simulink model "Project1"  (R2022b)
settings: Solver=VariableStepAuto  StartTime=0.0  StopTime=10.0  RelTol=1e-3
undefined symbols (not defined in the file): a, b, c
libraries: simulink x15
settings Model: Creator=ROYAN  LastModifiedBy=ROYAN

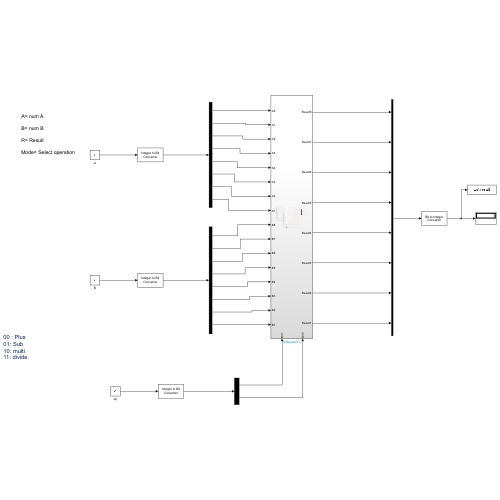
[thumbnail: Simulink's stored preview of the top-level diagram]
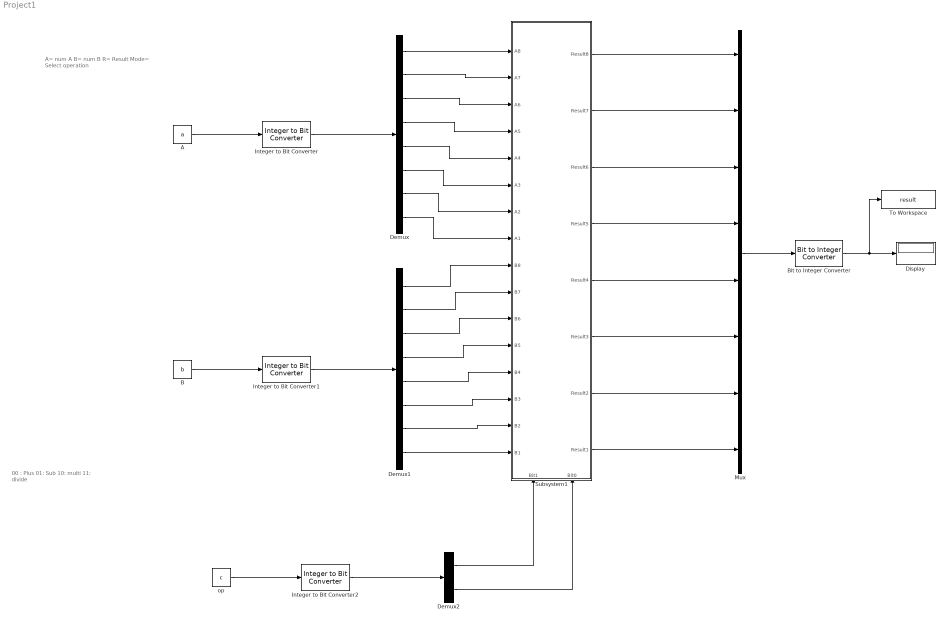
== system Project1 ==
  note: 00 : Plus
      | 01: Sub
      | 10: multi
      | 11: divide
  note: A= num A
      |
      | B= num B
      |
      | R= Result
      |
      | Mode= Select operation
  A : Constant  Value=a
  B : Constant  Value=b
  Bit to Integer Converter : simulink/Logic and Bit Operations/Bit to Integer Converter  nbits=8  bitOrder=MSB first  signedOutputValues=Signed  outDtype=Inherit via internal rule  outDtypeSigned=Inherit via internal rule
  Demux : Demux  Outputs=8
  Demux1 : Demux  Outputs=8
  Demux2 : Demux  Outputs=2
  Display : Display
  Integer to Bit Converter : simulink/Logic and Bit Operations/Integer to Bit Converter  nbits=8  signedInputValues=Unsigned  bitOrder=MSB first  outDtype=Inherit via internal rule
  Integer to Bit Converter1 : simulink/Logic and Bit Operations/Integer to Bit Converter  nbits=8  signedInputValues=Unsigned  bitOrder=MSB first  outDtype=Inherit via internal rule
  Integer to Bit Converter2 : simulink/Logic and Bit Operations/Integer to Bit Converter  nbits=2  signedInputValues=Unsigned  bitOrder=MSB first  outDtype=Inherit via internal rule
  Mux : Mux  Inputs=8
  Subsystem1 : Subsystem
      settings: PortSchema="{\"entries\":[{\"content\":{\"sides\":[{\"content\":{\"connectorIds\":[\"In1\",\"In2\",\"In3\",\"In4\",\"In5\",\"In6\",\"In7\",\"In8\",\"In9\",\"In10\",\"In11\",\"In12\",\"In13\",\"In14\",\"In15\",\"In16\"]},\"type\":\"ConnectorPlacement.EquallySpacedRectSide\",\"uuid\":\"3d59707f-8e10-42d7-a8bb-d15e440eb3d5\"},{\"content\":{\"connectorIds\":[\"Out1\",\"Out2\",\"Out3\",\"Out4\",\"Out5\",\"Out6\",\"Out7\",\"Out8\"],\"side\":\"RIGHT\"},\"type\":\"ConnectorPlacement.EquallySpacedRectSide\",\"uuid\":\"1a8263b8-a282-4efb-b962-f7f661c6be06\"},{\"content\":{\"connectorIds\":[],\"side\":\"TOP\"},\"type\":\"ConnectorPlacement.EquallySpacedRectSide\",\"uuid\":\"6e97006b-dc23-4e30-9819-71647844af05\"},{\"content\":{\"connectorIds\":[\"In17\",\"In18\"],\"side\":\"BOTTOM\"},\"type\":\"ConnectorPlacement.EquallySpacedRectSide\",\"uuid\":\"8a081856-ff6f-46be-8c16-ac5173067d34\"}]},\"type\":\"ConnectorPlacement.EquallySpacedConnector\",\"uuid\":\"19aafbc0-9711-4025-9e66-34128d3b56ae\"}],\"packageUris\":[\"http://schema.mathworks.com/mf0/Connector/R2020b\"],\"version\":\"1.0\"}"
  To Workspace : ToWorkspace  VariableName=result  SampleTime=-1
  op : Constant  Value=c
  wires:
  Subsystem1/1(Result8) -> Mux/1
  Subsystem1/2(Result7) -> Mux/2
  Subsystem1/3(Result6) -> Mux/3
  Subsystem1/4(Result5) -> Mux/4
  Subsystem1/7(Result2) -> Mux/7
  Subsystem1/8(Result1) -> Mux/8
  Subsystem1/6(Result3) -> Mux/6
  Subsystem1/5(Result4) -> Mux/5
  B/1 -> Integer to Bit Converter1/1
  Demux1/8 -> Subsystem1/16(B1)
  Demux1/7 -> Subsystem1/15(B2)
  Demux1/6 -> Subsystem1/14(B3)
  Demux1/5 -> Subsystem1/13(B4)
  Demux1/4 -> Subsystem1/12(B5)
  Mux/1 -> Bit to Integer Converter/1
  Bit to Integer Converter/1 -> To Workspace/1, Display/1
  Integer to Bit Converter1/1 -> Demux1/1
  Demux/1 -> Subsystem1/1(A8)
  Demux/2 -> Subsystem1/2(A7)
  Demux/3 -> Subsystem1/3(A6)
  Demux/4 -> Subsystem1/4(A5)
  Demux/5 -> Subsystem1/5(A4)
  Demux/6 -> Subsystem1/6(A3)
  Demux/7 -> Subsystem1/7(A2)
  Demux/8 -> Subsystem1/8(A1)
  Demux1/3 -> Subsystem1/11(B6)
  Demux1/1 -> Subsystem1/9(B8)
  Demux1/2 -> Subsystem1/10(B7)
  Integer to Bit Converter/1 -> Demux/1
  A/1 -> Integer to Bit Converter/1
  Integer to Bit Converter2/1 -> Demux2/1
  op/1 -> Integer to Bit Converter2/1
  Demux2/1 -> Subsystem1/17(Bit1)
  Demux2/2 -> Subsystem1/18(Bit0)

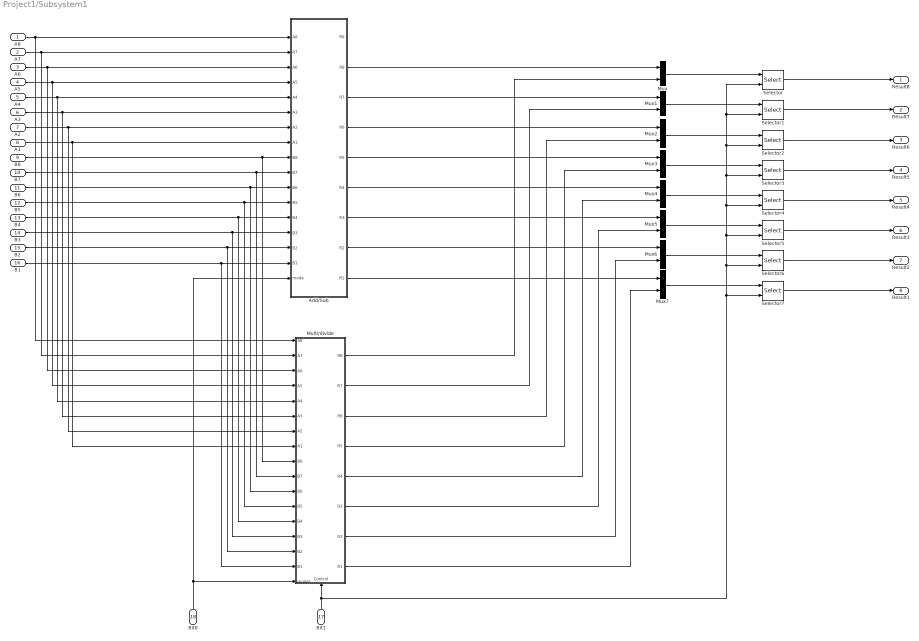
== system Project1/Subsystem1 ==
  A8 : Inport
  A7 : Inport  Port=2
  A6 : Inport  Port=3
  A5 : Inport  Port=4
  A4 : Inport  Port=5
  A3 : Inport  Port=6
  A2 : Inport  Port=7
  A1 : Inport  Port=8
  B8 : Inport  Port=9
  B7 : Inport  Port=10
  B6 : Inport  Port=11
  B5 : Inport  Port=12
  B4 : Inport  Port=13
  B3 : Inport  Port=14
  B2 : Inport  Port=15
  B1 : Inport  Port=16
  Bit1 : Inport  Port=17
  Bit0 : Inport  Port=18
  Add/Sub : Subsystem
  "Multi/divide " : Subsystem
      settings: PortSchema="{\"entries\":[{\"content\":{\"sides\":[{\"content\":{\"connectorIds\":[\"In1\",\"In2\",\"In3\",\"In4\",\"In5\",\"In6\",\"In7\",\"In8\",\"In9\",\"In10\",\"In11\",\"In12\",\"In13\",\"In14\",\"In15\",\"In16\",\"In17\"]},\"type\":\"ConnectorPlacement.EquallySpacedRectSide\",\"uuid\":\"d787903a-2fc8-4344-b2b5-b1474f8fa836\"},{\"content\":{\"connectorIds\":[\"Out1\",\"Out2\",\"Out3\",\"Out4\",\"Out5\",\"Out6\",\"Out7\",\"Out8\"],\"side\":\"RIGHT\"},\"type\":\"ConnectorPlacement.EquallySpacedRectSide\",\"uuid\":\"e4051a45-32f8-4700-a673-fbaf13b5a8eb\"},{\"content\":{\"connectorIds\":[],\"side\":\"TOP\"},\"type\":\"ConnectorPlacement.EquallySpacedRectSide\",\"uuid\":\"26f5a230-4be8-43df-bd8c-ec355ee08860\"},{\"content\":{\"connectorIds\":[\"In18\"],\"side\":\"BOTTOM\"},\"type\":\"ConnectorPlacement.EquallySpacedRectSide\",\"uuid\":\"cbf4e858-912e-4040-9d22-8fbb14c5758f\"}]},\"type\":\"ConnectorPlacement.EquallySpacedConnector\",\"uuid\":\"a4b69b5f-bd5b-46ed-959e-11d2f0394428\"}],\"packageUris\":[\"http://schema.mathworks.com/mf0/Connector/R2020b\"],\"version\":\"1.0\"}"
  Mux{,1..7} (8 alike) : Mux  Inputs=2
  Selector{,1..7} (8 alike) : Selector  NumberOfDimensions=2  IndexMode=Zero-based  InputPortWidth=3  IndexOptions=Select all,Index vector (port)  Indices=[1 3],1  OutputSizes=1,1
  Result8 : Outport
  Result7 : Outport  Port=2
  Result6 : Outport  Port=3
  Result5 : Outport  Port=4
  Result4 : Outport  Port=5
  Result3 : Outport  Port=6
  Result2 : Outport  Port=7
  Result1 : Outport  Port=8
  wires:
  A8/1 -> "Multi/divide "/1(A8), Add/Sub/1(A8)
  A7/1 -> "Multi/divide "/2(A7), Add/Sub/2(A7)
  A6/1 -> "Multi/divide "/3(A6), Add/Sub/3(A6)
  A5/1 -> "Multi/divide "/4(A5), Add/Sub/4(A5)
  A4/1 -> "Multi/divide "/5(A4), Add/Sub/5(A4)
  A3/1 -> "Multi/divide "/6(A3), Add/Sub/6(A3)
  A2/1 -> "Multi/divide "/7(A2), Add/Sub/7(A2)
  A1/1 -> "Multi/divide "/8(A1), Add/Sub/8(A1)
  B8/1 -> "Multi/divide "/9(B8), Add/Sub/9(B8)
  B7/1 -> "Multi/divide "/10(B7), Add/Sub/10(B7)
  B6/1 -> "Multi/divide "/11(B6), Add/Sub/11(B6)
  B5/1 -> "Multi/divide "/12(B5), Add/Sub/12(B5)
  B4/1 -> "Multi/divide "/13(B4), Add/Sub/13(B4)
  B3/1 -> "Multi/divide "/14(B3), Add/Sub/14(B3)
  B2/1 -> "Multi/divide "/15(B2), Add/Sub/15(B2)
  B1/1 -> "Multi/divide "/16(B1), Add/Sub/16(B1)
  Bit0/1 -> Add/Sub/17(mode), "Multi/divide "/17(mode1)
  Mux/1 -> Selector/1
  Selector/1 -> Result8/1
  Bit1/1 -> "Multi/divide "/18(Control), Selector6/2, Selector1/2, Selector/2, Selector2/2, Selector3/2, Selector4/2, Selector5/2, Selector7/2
  Selector1/1 -> Result7/1
  Mux1/1 -> Selector1/1
  Mux2/1 -> Selector2/1
  Selector2/1 -> Result6/1
  Mux3/1 -> Selector3/1
  Selector3/1 -> Result5/1
  Selector4/1 -> Result4/1
  Mux4/1 -> Selector4/1
  Mux5/1 -> Selector5/1
  Selector5/1 -> Result3/1
  Mux7/1 -> Selector7/1
  Mux6/1 -> Selector6/1
  Selector6/1 -> Result2/1
  Selector7/1 -> Result1/1
  Add/Sub/2(R8) -> Mux/1
  "Multi/divide "/1(R8) -> Mux/2
  Add/Sub/3(R7) -> Mux1/1
  "Multi/divide "/2(R7) -> Mux1/2
  Add/Sub/4(R6) -> Mux2/1
  "Multi/divide "/3(R6) -> Mux2/2
  Add/Sub/5(R5) -> Mux3/1
  "Multi/divide "/4(R5) -> Mux3/2
  Add/Sub/6(R4) -> Mux4/1
  "Multi/divide "/5(R4) -> Mux4/2
  Add/Sub/7(R3) -> Mux5/1
  "Multi/divide "/6(R3) -> Mux5/2
  Add/Sub/8(R2) -> Mux6/1
  "Multi/divide "/7(R2) -> Mux6/2
  Add/Sub/9(R1) -> Mux7/1
  "Multi/divide "/8(R1) -> Mux7/2

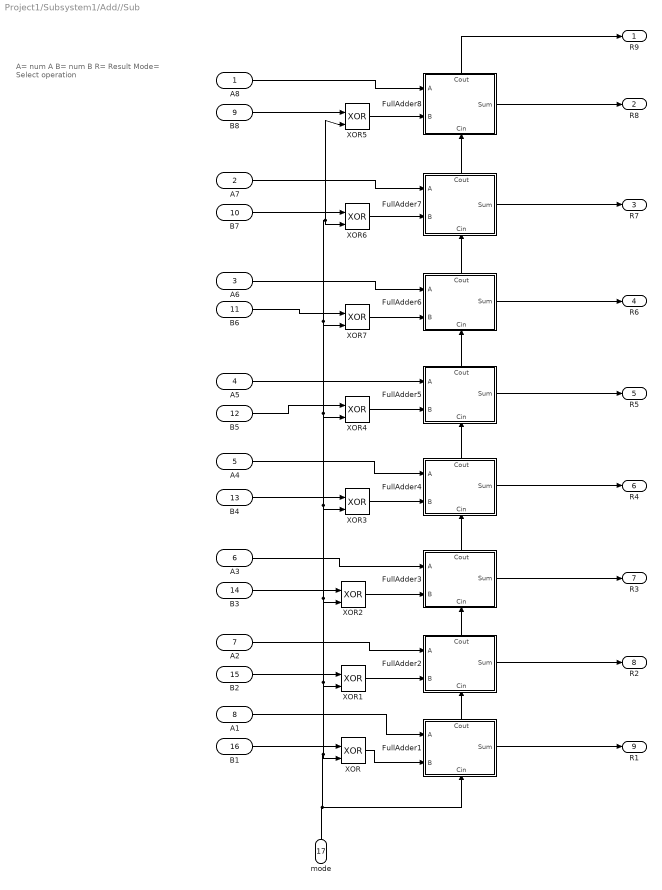
== system Project1/Subsystem1/Add//Sub ==
  note: A= num A
      |
      | B= num B
      |
      | R= Result
      |
      | Mode= Select operation
  A8 : Inport
  A7 : Inport  Port=2
  A6 : Inport  Port=3
  A5 : Inport  Port=4
  A4 : Inport  Port=5
  A3 : Inport  Port=6
  A2 : Inport  Port=7
  A1 : Inport  Port=8
  B8 : Inport  Port=9
  B7 : Inport  Port=10
  B6 : Inport  Port=11
  B5 : Inport  Port=12
  B4 : Inport  Port=13
  B3 : Inport  Port=14
  B2 : Inport  Port=15
  B1 : Inport  Port=16
  mode : Inport  Port=17
  FullAdder1 : Subsystem
      settings: PortSchema="{\"entries\":[{\"content\":{\"sides\":[{\"content\":{\"connectorIds\":[\"In1\",\"In2\"]},\"type\":\"ConnectorPlacement.EquallySpacedRectSide\",\"uuid\":\"fe566a19-caaa-40f2-a564-acf59556d540\"},{\"content\":{\"connectorIds\":[\"Out1\"],\"side\":\"RIGHT\"},\"type\":\"ConnectorPlacement.EquallySpacedRectSide\",\"uuid\":\"72e5ab5f-929d-480e-bf59-fcaf5ea21c8f\"},{\"content\":{\"connectorIds\":[\"Out2\"],\"side\":\"TOP\"},\"type\":\"ConnectorPlacement.EquallySpacedRectSide\",\"uuid\":\"fa7afc02-c581-4624-b2e4-f0b490a4f45a\"},{\"content\":{\"connectorIds\":[\"In3\"],\"side\":\"BOTTOM\"},\"type\":\"ConnectorPlacement.EquallySpacedRectSide\",\"uuid\":\"7004099e-9eda-49bf-b4e1-5ef4db972604\"}]},\"type\":\"ConnectorPlacement.EquallySpacedConnector\",\"uuid\":\"f3081cfd-4ff5-48bf-a714-5b2ae9791e36\"}],\"packageUris\":[\"http://schema.mathworks.com/mf0/Connector/R2020b\"],\"version\":\"1.0\"}"
  FullAdder2 : Subsystem
      settings: PortSchema="{\"entries\":[{\"content\":{\"sides\":[{\"content\":{\"connectorIds\":[\"In1\",\"In2\"]},\"type\":\"ConnectorPlacement.EquallySpacedRectSide\",\"uuid\":\"fe566a19-caaa-40f2-a564-acf59556d540\"},{\"content\":{\"connectorIds\":[\"Out1\"],\"side\":\"RIGHT\"},\"type\":\"ConnectorPlacement.EquallySpacedRectSide\",\"uuid\":\"72e5ab5f-929d-480e-bf59-fcaf5ea21c8f\"},{\"content\":{\"connectorIds\":[\"Out2\"],\"side\":\"TOP\"},\"type\":\"ConnectorPlacement.EquallySpacedRectSide\",\"uuid\":\"fa7afc02-c581-4624-b2e4-f0b490a4f45a\"},{\"content\":{\"connectorIds\":[\"In3\"],\"side\":\"BOTTOM\"},\"type\":\"ConnectorPlacement.EquallySpacedRectSide\",\"uuid\":\"7004099e-9eda-49bf-b4e1-5ef4db972604\"}]},\"type\":\"ConnectorPlacement.EquallySpacedConnector\",\"uuid\":\"f3081cfd-4ff5-48bf-a714-5b2ae9791e36\"}],\"packageUris\":[\"http://schema.mathworks.com/mf0/Connector/R2020b\"],\"version\":\"1.0\"}"
  FullAdder3 : Subsystem
      settings: PortSchema="{\"entries\":[{\"content\":{\"sides\":[{\"content\":{\"connectorIds\":[\"In1\",\"In2\"]},\"type\":\"ConnectorPlacement.EquallySpacedRectSide\",\"uuid\":\"fe566a19-caaa-40f2-a564-acf59556d540\"},{\"content\":{\"connectorIds\":[\"Out1\"],\"side\":\"RIGHT\"},\"type\":\"ConnectorPlacement.EquallySpacedRectSide\",\"uuid\":\"72e5ab5f-929d-480e-bf59-fcaf5ea21c8f\"},{\"content\":{\"connectorIds\":[\"Out2\"],\"side\":\"TOP\"},\"type\":\"ConnectorPlacement.EquallySpacedRectSide\",\"uuid\":\"fa7afc02-c581-4624-b2e4-f0b490a4f45a\"},{\"content\":{\"connectorIds\":[\"In3\"],\"side\":\"BOTTOM\"},\"type\":\"ConnectorPlacement.EquallySpacedRectSide\",\"uuid\":\"7004099e-9eda-49bf-b4e1-5ef4db972604\"}]},\"type\":\"ConnectorPlacement.EquallySpacedConnector\",\"uuid\":\"f3081cfd-4ff5-48bf-a714-5b2ae9791e36\"}],\"packageUris\":[\"http://schema.mathworks.com/mf0/Connector/R2020b\"],\"version\":\"1.0\"}"
  FullAdder4 : Subsystem
      settings: PortSchema="{\"entries\":[{\"content\":{\"sides\":[{\"content\":{\"connectorIds\":[\"In1\",\"In2\"]},\"type\":\"ConnectorPlacement.EquallySpacedRectSide\",\"uuid\":\"fe566a19-caaa-40f2-a564-acf59556d540\"},{\"content\":{\"connectorIds\":[\"Out1\"],\"side\":\"RIGHT\"},\"type\":\"ConnectorPlacement.EquallySpacedRectSide\",\"uuid\":\"72e5ab5f-929d-480e-bf59-fcaf5ea21c8f\"},{\"content\":{\"connectorIds\":[\"Out2\"],\"side\":\"TOP\"},\"type\":\"ConnectorPlacement.EquallySpacedRectSide\",\"uuid\":\"fa7afc02-c581-4624-b2e4-f0b490a4f45a\"},{\"content\":{\"connectorIds\":[\"In3\"],\"side\":\"BOTTOM\"},\"type\":\"ConnectorPlacement.EquallySpacedRectSide\",\"uuid\":\"7004099e-9eda-49bf-b4e1-5ef4db972604\"}]},\"type\":\"ConnectorPlacement.EquallySpacedConnector\",\"uuid\":\"f3081cfd-4ff5-48bf-a714-5b2ae9791e36\"}],\"packageUris\":[\"http://schema.mathworks.com/mf0/Connector/R2020b\"],\"version\":\"1.0\"}"
  FullAdder5 : Subsystem
      settings: PortSchema="{\"entries\":[{\"content\":{\"sides\":[{\"content\":{\"connectorIds\":[\"In1\",\"In2\"]},\"type\":\"ConnectorPlacement.EquallySpacedRectSide\",\"uuid\":\"fe566a19-caaa-40f2-a564-acf59556d540\"},{\"content\":{\"connectorIds\":[\"Out1\"],\"side\":\"RIGHT\"},\"type\":\"ConnectorPlacement.EquallySpacedRectSide\",\"uuid\":\"72e5ab5f-929d-480e-bf59-fcaf5ea21c8f\"},{\"content\":{\"connectorIds\":[\"Out2\"],\"side\":\"TOP\"},\"type\":\"ConnectorPlacement.EquallySpacedRectSide\",\"uuid\":\"fa7afc02-c581-4624-b2e4-f0b490a4f45a\"},{\"content\":{\"connectorIds\":[\"In3\"],\"side\":\"BOTTOM\"},\"type\":\"ConnectorPlacement.EquallySpacedRectSide\",\"uuid\":\"7004099e-9eda-49bf-b4e1-5ef4db972604\"}]},\"type\":\"ConnectorPlacement.EquallySpacedConnector\",\"uuid\":\"f3081cfd-4ff5-48bf-a714-5b2ae9791e36\"}],\"packageUris\":[\"http://schema.mathworks.com/mf0/Connector/R2020b\"],\"version\":\"1.0\"}"
  FullAdder6 : Subsystem
      settings: PortSchema="{\"entries\":[{\"content\":{\"sides\":[{\"content\":{\"connectorIds\":[\"In1\",\"In2\"]},\"type\":\"ConnectorPlacement.EquallySpacedRectSide\",\"uuid\":\"fe566a19-caaa-40f2-a564-acf59556d540\"},{\"content\":{\"connectorIds\":[\"Out1\"],\"side\":\"RIGHT\"},\"type\":\"ConnectorPlacement.EquallySpacedRectSide\",\"uuid\":\"72e5ab5f-929d-480e-bf59-fcaf5ea21c8f\"},{\"content\":{\"connectorIds\":[\"Out2\"],\"side\":\"TOP\"},\"type\":\"ConnectorPlacement.EquallySpacedRectSide\",\"uuid\":\"fa7afc02-c581-4624-b2e4-f0b490a4f45a\"},{\"content\":{\"connectorIds\":[\"In3\"],\"side\":\"BOTTOM\"},\"type\":\"ConnectorPlacement.EquallySpacedRectSide\",\"uuid\":\"7004099e-9eda-49bf-b4e1-5ef4db972604\"}]},\"type\":\"ConnectorPlacement.EquallySpacedConnector\",\"uuid\":\"f3081cfd-4ff5-48bf-a714-5b2ae9791e36\"}],\"packageUris\":[\"http://schema.mathworks.com/mf0/Connector/R2020b\"],\"version\":\"1.0\"}"
  FullAdder7 : Subsystem
      settings: PortSchema="{\"entries\":[{\"content\":{\"sides\":[{\"content\":{\"connectorIds\":[\"In1\",\"In2\"]},\"type\":\"ConnectorPlacement.EquallySpacedRectSide\",\"uuid\":\"fe566a19-caaa-40f2-a564-acf59556d540\"},{\"content\":{\"connectorIds\":[\"Out1\"],\"side\":\"RIGHT\"},\"type\":\"ConnectorPlacement.EquallySpacedRectSide\",\"uuid\":\"72e5ab5f-929d-480e-bf59-fcaf5ea21c8f\"},{\"content\":{\"connectorIds\":[\"Out2\"],\"side\":\"TOP\"},\"type\":\"ConnectorPlacement.EquallySpacedRectSide\",\"uuid\":\"fa7afc02-c581-4624-b2e4-f0b490a4f45a\"},{\"content\":{\"connectorIds\":[\"In3\"],\"side\":\"BOTTOM\"},\"type\":\"ConnectorPlacement.EquallySpacedRectSide\",\"uuid\":\"7004099e-9eda-49bf-b4e1-5ef4db972604\"}]},\"type\":\"ConnectorPlacement.EquallySpacedConnector\",\"uuid\":\"f3081cfd-4ff5-48bf-a714-5b2ae9791e36\"}],\"packageUris\":[\"http://schema.mathworks.com/mf0/Connector/R2020b\"],\"version\":\"1.0\"}"
  FullAdder8 : Subsystem
      settings: PortSchema="{\"entries\":[{\"content\":{\"sides\":[{\"content\":{\"connectorIds\":[\"In1\",\"In2\"]},\"type\":\"ConnectorPlacement.EquallySpacedRectSide\",\"uuid\":\"fe566a19-caaa-40f2-a564-acf59556d540\"},{\"content\":{\"connectorIds\":[\"Out1\"],\"side\":\"RIGHT\"},\"type\":\"ConnectorPlacement.EquallySpacedRectSide\",\"uuid\":\"72e5ab5f-929d-480e-bf59-fcaf5ea21c8f\"},{\"content\":{\"connectorIds\":[\"Out2\"],\"side\":\"TOP\"},\"type\":\"ConnectorPlacement.EquallySpacedRectSide\",\"uuid\":\"fa7afc02-c581-4624-b2e4-f0b490a4f45a\"},{\"content\":{\"connectorIds\":[\"In3\"],\"side\":\"BOTTOM\"},\"type\":\"ConnectorPlacement.EquallySpacedRectSide\",\"uuid\":\"7004099e-9eda-49bf-b4e1-5ef4db972604\"}]},\"type\":\"ConnectorPlacement.EquallySpacedConnector\",\"uuid\":\"f3081cfd-4ff5-48bf-a714-5b2ae9791e36\"}],\"packageUris\":[\"http://schema.mathworks.com/mf0/Connector/R2020b\"],\"version\":\"1.0\"}"
  XOR{,1..7} (8 alike) : Logic  Operator=XOR  IconShape=distinctive  AllPortsSameDT=off  OutDataTypeStr=boolean
  R9 : Outport
  R8 : Outport  Port=2
  R7 : Outport  Port=3
  R6 : Outport  Port=4
  R5 : Outport  Port=5
  R4 : Outport  Port=6
  R3 : Outport  Port=7
  R2 : Outport  Port=8
  R1 : Outport  Port=9
  wires:
  FullAdder1/2(Cout) -> FullAdder2/3(Cin)
  FullAdder3/2(Cout) -> FullAdder4/3(Cin)
  A6/1 -> FullAdder6/1(A)
  FullAdder3/1(Sum) -> R3/1
  FullAdder6/2(Cout) -> FullAdder7/3(Cin)
  FullAdder5/2(Cout) -> FullAdder6/3(Cin)
  FullAdder1/1(Sum) -> R1/1
  A8/1 -> FullAdder8/1(A)
  FullAdder8/1(Sum) -> R8/1
  FullAdder5/1(Sum) -> R5/1
  A7/1 -> FullAdder7/1(A)
  A5/1 -> FullAdder5/1(A)
  FullAdder4/2(Cout) -> FullAdder5/3(Cin)
  FullAdder4/1(Sum) -> R4/1
  FullAdder6/1(Sum) -> R6/1
  A2/1 -> FullAdder2/1(A)
  FullAdder8/2(Cout) -> R9/1
  A4/1 -> FullAdder4/1(A)
  FullAdder2/1(Sum) -> R2/1
  FullAdder7/2(Cout) -> FullAdder8/3(Cin)
  A1/1 -> FullAdder1/1(A)
  A3/1 -> FullAdder3/1(A)
  FullAdder2/2(Cout) -> FullAdder3/3(Cin)
  FullAdder7/1(Sum) -> R7/1
  mode/1 -> XOR5/2, XOR6/2, XOR7/2, XOR4/2, XOR3/2, XOR2/2, XOR1/2, XOR/2, FullAdder1/3(Cin)
  B1/1 -> XOR/1
  XOR/1 -> FullAdder1/2(B)
  B2/1 -> XOR1/1
  XOR1/1 -> FullAdder2/2(B)
  B3/1 -> XOR2/1
  XOR2/1 -> FullAdder3/2(B)
  B4/1 -> XOR3/1
  XOR3/1 -> FullAdder4/2(B)
  B5/1 -> XOR4/1
  XOR4/1 -> FullAdder5/2(B)
  B6/1 -> XOR7/1
  XOR7/1 -> FullAdder6/2(B)
  B7/1 -> XOR6/1
  XOR6/1 -> FullAdder7/2(B)
  B8/1 -> XOR5/1
  XOR5/1 -> FullAdder8/2(B)

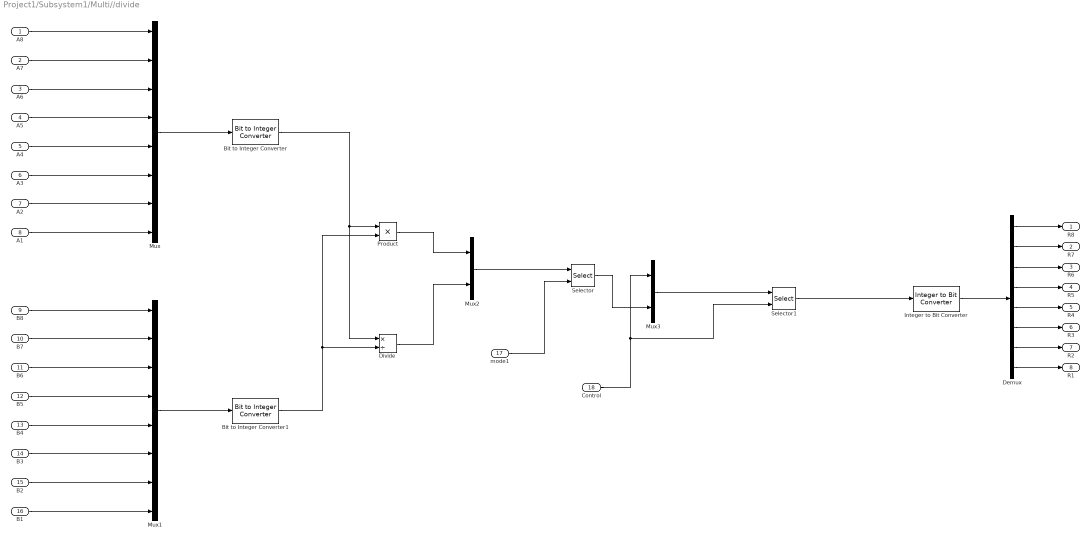
== system Project1/Subsystem1/Multi//divide  ==
  A8 : Inport
  A7 : Inport  Port=2
  A6 : Inport  Port=3
  A5 : Inport  Port=4
  A4 : Inport  Port=5
  A3 : Inport  Port=6
  A2 : Inport  Port=7
  A1 : Inport  Port=8
  B8 : Inport  Port=9
  B7 : Inport  Port=10
  B6 : Inport  Port=11
  B5 : Inport  Port=12
  B4 : Inport  Port=13
  B3 : Inport  Port=14
  B2 : Inport  Port=15
  B1 : Inport  Port=16
  mode1 : Inport  Port=17
  Control : Inport  Port=18
  Bit to Integer Converter : simulink/Logic and Bit Operations/Bit to Integer Converter  nbits=8  bitOrder=MSB first  signedOutputValues=Unsigned  outDtype=Inherit via internal rule  outDtypeSigned=Inherit via internal rule
  Bit to Integer Converter1 : simulink/Logic and Bit Operations/Bit to Integer Converter  nbits=8  bitOrder=MSB first  signedOutputValues=Unsigned  outDtype=Inherit via internal rule  outDtypeSigned=Inherit via internal rule
  Demux : Demux  Outputs=8
  Divide : Product  Inputs=*/
  Integer to Bit Converter : simulink/Logic and Bit Operations/Integer to Bit Converter  nbits=8  signedInputValues=Unsigned  bitOrder=MSB first  outDtype=Inherit via internal rule
  Mux : Mux  Inputs=8
  Mux1 : Mux  Inputs=8
  Mux2 : Mux  Inputs=2
  Mux3 : Mux  Inputs=2
  Product : Product
  Selector : Selector  NumberOfDimensions=2  IndexMode=Zero-based  InputPortWidth=3  IndexOptions=Select all,Index vector (port)  Indices=[1 3],1  OutputSizes=1,1
  Selector1 : Selector  NumberOfDimensions=2  IndexMode=Zero-based  InputPortWidth=3  IndexOptions=Select all,Index vector (port)  Indices=[1 3],1  OutputSizes=1,1
  R8 : Outport
  R7 : Outport  Port=2
  R6 : Outport  Port=3
  R5 : Outport  Port=4
  R4 : Outport  Port=5
  R3 : Outport  Port=6
  R2 : Outport  Port=7
  R1 : Outport  Port=8
  wires:
  A8/1 -> Mux/1
  A7/1 -> Mux/2
  A6/1 -> Mux/3
  A5/1 -> Mux/4
  A4/1 -> Mux/5
  A2/1 -> Mux/7
  A1/1 -> Mux/8
  A3/1 -> Mux/6
  Mux/1 -> Bit to Integer Converter/1
  Mux1/1 -> Bit to Integer Converter1/1
  B8/1 -> Mux1/1
  B7/1 -> Mux1/2
  B6/1 -> Mux1/3
  B5/1 -> Mux1/4
  B4/1 -> Mux1/5
  B3/1 -> Mux1/6
  B2/1 -> Mux1/7
  B1/1 -> Mux1/8
  Bit to Integer Converter/1 -> Divide/1, Product/1
  Bit to Integer Converter1/1 -> Product/2, Divide/2
  Product/1 -> Mux2/1
  Divide/1 -> Mux2/2
  mode1/1 -> Selector/2
  Mux2/1 -> Selector/1
  Integer to Bit Converter/1 -> Demux/1
  Demux/1 -> R8/1
  Demux/2 -> R7/1
  Demux/8 -> R1/1
  Demux/7 -> R2/1
  Demux/6 -> R3/1
  Demux/5 -> R4/1
  Demux/4 -> R5/1
  Demux/3 -> R6/1
  Control/1 -> Mux3/1, Selector1/2
  Selector1/1 -> Integer to Bit Converter/1
  Mux3/1 -> Selector1/1
  Selector/1 -> Mux3/2

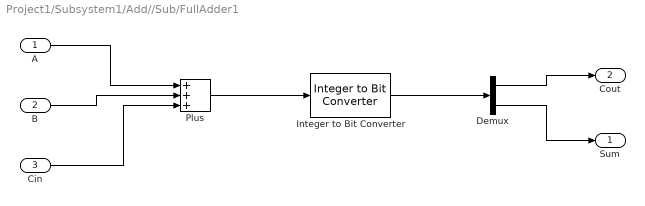
== system Project1/Subsystem1/Add//Sub/FullAdder1 ==
  A : Inport
  B : Inport  Port=2
  Cin : Inport  Port=3
  Demux : Demux  Outputs=2
  Integer to Bit Converter : simulink/Logic and Bit Operations/Integer to Bit Converter  nbits=2  signedInputValues=Unsigned  bitOrder=MSB first  outDtype=Inherit via internal rule
  Plus : Sum  Inputs=+++
  Sum : Outport
  Cout : Outport  Port=2
  wires:
  Demux/2 -> Sum/1
  Demux/1 -> Cout/1
  A/1 -> Plus/1
  Cin/1 -> Plus/3
  Plus/1 -> Integer to Bit Converter/1
  B/1 -> Plus/2
  Integer to Bit Converter/1 -> Demux/1

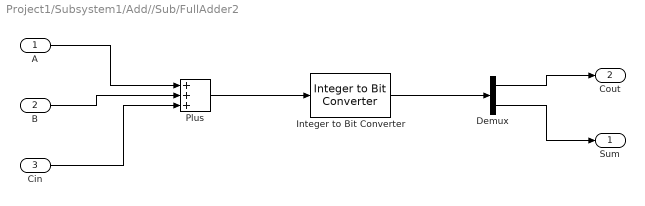
== system Project1/Subsystem1/Add//Sub/FullAdder2 ==
  A : Inport
  B : Inport  Port=2
  Cin : Inport  Port=3
  Demux : Demux  Outputs=2
  Integer to Bit Converter : simulink/Logic and Bit Operations/Integer to Bit Converter  nbits=2  signedInputValues=Unsigned  bitOrder=MSB first  outDtype=Inherit via internal rule
  Plus : Sum  Inputs=+++
  Sum : Outport
  Cout : Outport  Port=2
  wires:
  Demux/2 -> Sum/1
  Demux/1 -> Cout/1
  A/1 -> Plus/1
  Cin/1 -> Plus/3
  Plus/1 -> Integer to Bit Converter/1
  B/1 -> Plus/2
  Integer to Bit Converter/1 -> Demux/1

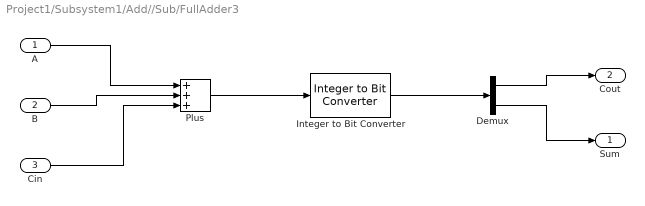
== system Project1/Subsystem1/Add//Sub/FullAdder3 ==
  A : Inport
  B : Inport  Port=2
  Cin : Inport  Port=3
  Demux : Demux  Outputs=2
  Integer to Bit Converter : simulink/Logic and Bit Operations/Integer to Bit Converter  nbits=2  signedInputValues=Unsigned  bitOrder=MSB first  outDtype=Inherit via internal rule
  Plus : Sum  Inputs=+++
  Sum : Outport
  Cout : Outport  Port=2
  wires:
  Integer to Bit Converter/1 -> Demux/1
  B/1 -> Plus/2
  Plus/1 -> Integer to Bit Converter/1
  Cin/1 -> Plus/3
  A/1 -> Plus/1
  Demux/1 -> Cout/1
  Demux/2 -> Sum/1

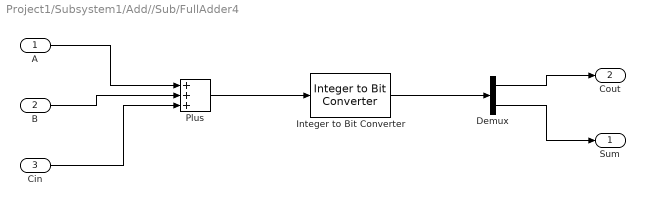
== system Project1/Subsystem1/Add//Sub/FullAdder4 ==
  A : Inport
  B : Inport  Port=2
  Cin : Inport  Port=3
  Demux : Demux  Outputs=2
  Integer to Bit Converter : simulink/Logic and Bit Operations/Integer to Bit Converter  nbits=2  signedInputValues=Unsigned  bitOrder=MSB first  outDtype=Inherit via internal rule
  Plus : Sum  Inputs=+++
  Sum : Outport
  Cout : Outport  Port=2
  wires:
  Demux/2 -> Sum/1
  Demux/1 -> Cout/1
  A/1 -> Plus/1
  Cin/1 -> Plus/3
  Plus/1 -> Integer to Bit Converter/1
  B/1 -> Plus/2
  Integer to Bit Converter/1 -> Demux/1

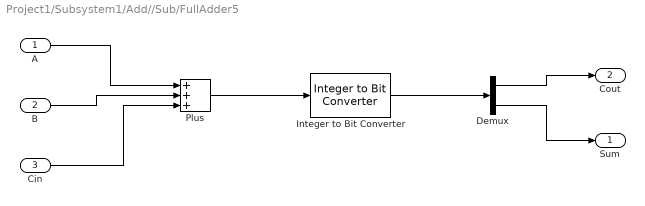
== system Project1/Subsystem1/Add//Sub/FullAdder5 ==
  A : Inport
  B : Inport  Port=2
  Cin : Inport  Port=3
  Demux : Demux  Outputs=2
  Integer to Bit Converter : simulink/Logic and Bit Operations/Integer to Bit Converter  nbits=2  signedInputValues=Unsigned  bitOrder=MSB first  outDtype=Inherit via internal rule
  Plus : Sum  Inputs=+++
  Sum : Outport
  Cout : Outport  Port=2
  wires:
  Integer to Bit Converter/1 -> Demux/1
  B/1 -> Plus/2
  Plus/1 -> Integer to Bit Converter/1
  Cin/1 -> Plus/3
  A/1 -> Plus/1
  Demux/1 -> Cout/1
  Demux/2 -> Sum/1

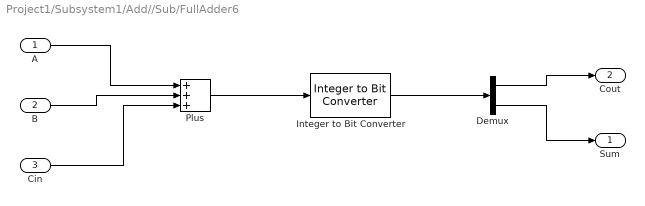
== system Project1/Subsystem1/Add//Sub/FullAdder6 ==
  A : Inport
  B : Inport  Port=2
  Cin : Inport  Port=3
  Demux : Demux  Outputs=2
  Integer to Bit Converter : simulink/Logic and Bit Operations/Integer to Bit Converter  nbits=2  signedInputValues=Unsigned  bitOrder=MSB first  outDtype=Inherit via internal rule
  Plus : Sum  Inputs=+++
  Sum : Outport
  Cout : Outport  Port=2
  wires:
  Demux/2 -> Sum/1
  Demux/1 -> Cout/1
  A/1 -> Plus/1
  Cin/1 -> Plus/3
  Plus/1 -> Integer to Bit Converter/1
  B/1 -> Plus/2
  Integer to Bit Converter/1 -> Demux/1

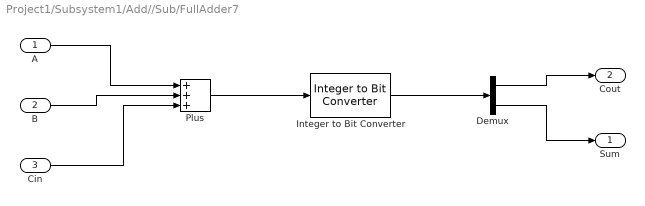
== system Project1/Subsystem1/Add//Sub/FullAdder7 ==
  A : Inport
  B : Inport  Port=2
  Cin : Inport  Port=3
  Demux : Demux  Outputs=2
  Integer to Bit Converter : simulink/Logic and Bit Operations/Integer to Bit Converter  nbits=2  signedInputValues=Unsigned  bitOrder=MSB first  outDtype=Inherit via internal rule
  Plus : Sum  Inputs=+++
  Sum : Outport
  Cout : Outport  Port=2
  wires:
  Integer to Bit Converter/1 -> Demux/1
  B/1 -> Plus/2
  Plus/1 -> Integer to Bit Converter/1
  Cin/1 -> Plus/3
  A/1 -> Plus/1
  Demux/1 -> Cout/1
  Demux/2 -> Sum/1

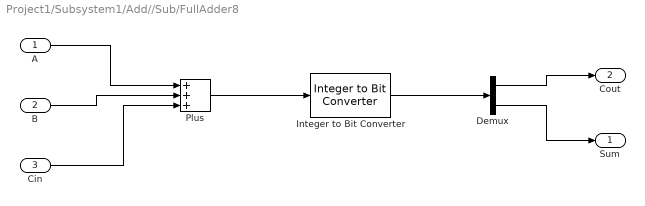
== system Project1/Subsystem1/Add//Sub/FullAdder8 ==
  A : Inport
  B : Inport  Port=2
  Cin : Inport  Port=3
  Demux : Demux  Outputs=2
  Integer to Bit Converter : simulink/Logic and Bit Operations/Integer to Bit Converter  nbits=2  signedInputValues=Unsigned  bitOrder=MSB first  outDtype=Inherit via internal rule
  Plus : Sum  Inputs=+++
  Sum : Outport
  Cout : Outport  Port=2
  wires:
  Demux/2 -> Sum/1
  Demux/1 -> Cout/1
  A/1 -> Plus/1
  Cin/1 -> Plus/3
  Plus/1 -> Integer to Bit Converter/1
  B/1 -> Plus/2
  Integer to Bit Converter/1 -> Demux/1
